simulink model "grading"  (R2021b)
settings: Solver=VariableStepAuto  StartTime=0.0  StopTime=10.0  RelTol=1e-3
settings Model: Creator=midol  LastModifiedBy=midol

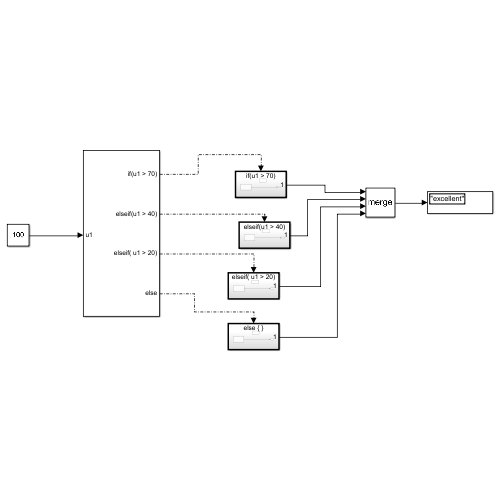
[thumbnail: Simulink's stored preview of the top-level diagram]
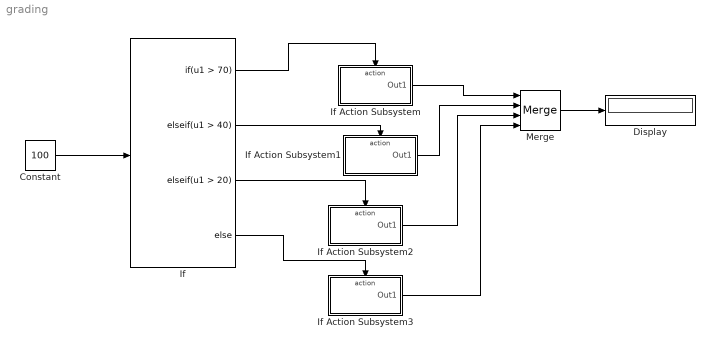
== system grading ==
  Constant : Constant  Value=100
  Display : Display
  If : If  IfExpression=u1 > 70  ElseIfExpressions=u1 > 40, u1 > 20
  If Action Subsystem : Subsystem  TreatAsAtomicUnit=on
  If Action Subsystem1 : Subsystem  TreatAsAtomicUnit=on
  If Action Subsystem2 : Subsystem  TreatAsAtomicUnit=on
  If Action Subsystem3 : Subsystem  TreatAsAtomicUnit=on
  Merge : Merge  Inputs=4
  wires:
  If/1 -> If Action Subsystem/Action
  If/2 -> If Action Subsystem1/Action
  If/3 -> If Action Subsystem2/Action
  If/4 -> If Action Subsystem3/Action
  Constant/1 -> If/1
  If Action Subsystem/1(Out1) -> Merge/1
  If Action Subsystem1/1(Out1) -> Merge/2
  If Action Subsystem2/1(Out1) -> Merge/3
  If Action Subsystem3/1(Out1) -> Merge/4
  Merge/1 -> Display/1

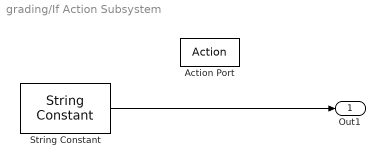
== system grading/If Action Subsystem ==
  Action Port : ActionPort  ActionPortLabel=if(u1 > 70)
  String Constant : StringConstant  String="\"excellent\""
  Out1 : Outport
  wires:
  String Constant/1 -> Out1/1

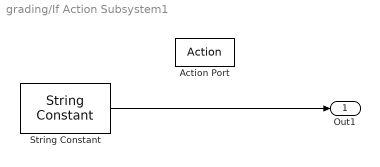
== system grading/If Action Subsystem1 ==
  Action Port : ActionPort  ActionPortLabel=elseif(u1 > 40)
  String Constant : StringConstant  String="\"very good\""
  Out1 : Outport
  wires:
  String Constant/1 -> Out1/1

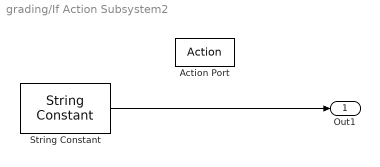
== system grading/If Action Subsystem2 ==
  Action Port : ActionPort  ActionPortLabel=elseif( u1 > 20)
  String Constant : StringConstant  String="\"pass\""
  Out1 : Outport
  wires:
  String Constant/1 -> Out1/1

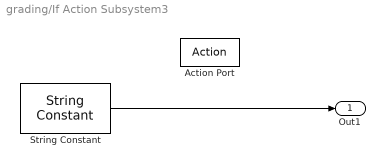
== system grading/If Action Subsystem3 ==
  Action Port : ActionPort  ActionPortLabel=else
  String Constant : StringConstant  String="\"fail\""
  Out1 : Outport
  wires:
  String Constant/1 -> Out1/1
